simulink model "external_state_machine"  (R2021a)
settings: Solver=FixedStepDiscrete  StartTime=0.0  StopTime=2000*t_ADC  RelTol=1e-3
values from neighbouring files (symbols this model uses):
  A = 0.1    [uz_mpc_6ph_init.m]    (also in uz_mpc_6ph_state_machine_init.m)
  IB = sqrt(2)*IR    [uz_mpc_6ph_init.m]    (also in uz_mpc_6ph_state_machine_init.m)
  id_ref = 0.0    (= 0)    [uz_mpc_6ph_init.m]    (also in uz_mpc_6ph_state_machine_init.m)
  iq_ref = 15.0    (= 15)    [uz_mpc_6ph_init.m]    (also in uz_mpc_6ph_state_machine_init.m = 10)
  ix_ref = 0.0    (= 0)    [uz_mpc_6ph_init.m]    (also in uz_mpc_6ph_state_machine_init.m)
  iy_ref = 0.0    (= 0)    [uz_mpc_6ph_init.m]    (also in uz_mpc_6ph_state_machine_init.m)
  lambda_d = 1.0    (= 1)    [uz_mpc_6ph_init.m]    (also in uz_mpc_6ph_state_machine_init.m)
  lambda_q = 1.0    (= 1)    [uz_mpc_6ph_init.m]    (also in uz_mpc_6ph_state_machine_init.m)
  lambda_u = 0.0    (= 0)    [uz_mpc_6ph_init.m]    (also in uz_mpc_6ph_state_machine_init.m)
  lambda_x = 1.0    (= 1)    [uz_mpc_6ph_init.m]    (also in uz_mpc_6ph_state_machine_init.m)
  lambda_y = 1.0    (= 1)    [uz_mpc_6ph_init.m]    (also in uz_mpc_6ph_state_machine_init.m)
  Ld_over_LB = Ld/LB    [uz_mpc_6ph_init.m]    (also in uz_mpc_6ph_state_machine_init.m)
  Lq_over_LB = Lq/LB    [uz_mpc_6ph_init.m]    (also in uz_mpc_6ph_state_machine_init.m)
  n_rpm = 2200.0    (= 2200)    [uz_mpc_6ph_init.m]    (also in uz_mpc_6ph_state_machine_init.m = 100)
  omega_m = n_rpm*pi/30    (= 230.383461263)    [uz_mpc_6ph_init.m]    (also in uz_mpc_6ph_state_machine_init.m = 10.471975512)
  omegaB = nR*2*pi()/60*p    [uz_mpc_6ph_init.m]    (also in uz_mpc_6ph_state_machine_init.m)
  p = 5    [uz_mpc_6ph_init.m]    (also in uz_mpc_6ph_state_machine_init.m)
  psi_pm_over_psiB = psi_pm/psiB    [uz_mpc_6ph_init.m]    (also in uz_mpc_6ph_state_machine_init.m)
  Rs_over_ZB = Rs/ZB    [uz_mpc_6ph_init.m]    (also in uz_mpc_6ph_state_machine_init.m)
  t_ADC = 1/f_ADC    (= 1e-05)    [uz_mpc_6ph_init.m]    (also in uz_mpc_6ph_state_machine_init.m)
  t_clock = 1/f_clock    (= 1e-08)    [uz_mpc_6ph_init.m]    (also in uz_mpc_6ph_state_machine_init.m)
  Ts_times_ZB_over_Ld = Ts*ZB/Ld    [uz_mpc_6ph_init.m]    (also in uz_mpc_6ph_state_machine_init.m)
  Ts_times_ZB_over_Lq = Ts*ZB/Lq    [uz_mpc_6ph_init.m]    (also in uz_mpc_6ph_state_machine_init.m)
  Ts_times_ZB_over_Lx = Ts*ZB/Lx    [uz_mpc_6ph_init.m]    (also in uz_mpc_6ph_state_machine_init.m)
  Ts_times_ZB_over_Ly = Ts*ZB/Ly    [uz_mpc_6ph_init.m]    (also in uz_mpc_6ph_state_machine_init.m)
  v_dc = 565.0    (= 565)    [uz_mpc_6ph_init.m]    (also in uz_mpc_6ph_state_machine_init.m = 50)
  VB = sqrt(2/3)*VR    [uz_mpc_6ph_init.m]    (also in uz_mpc_6ph_state_machine_init.m)
libraries: nesl_utility x38, fl_lib x30, simulink x19, ee_lib x14, hdlsllib x4, spsAlphaBetaZerotodq0Lib x1
(part 4 of 4)

== matlab function external_state_machine/uz_vsd_6ph_30deg/VSD_6ph_30deg ==
  settings: fimath=fimath('RoundingMethod', 'Floor','OverflowAction', 'Wrap','ProductMode', 'FullPrecision', 'SumMode', 'FullPrecision')
  data: a1 input; alpha output; b1 input; c1 input; a2 input; b2 input; c2 input; beta output; x1 output; y1 output; z1 output; z2 output
function [alpha,beta,x1,y1,z1,z2] = fcn(a1,b1,c1,a2,b2,c2)


A = [fi(0,1,18,11) fi(0,1,18,11) fi(0,1,18,11) fi(0,1,18,11) fi(0,1,18,11) fi(0,1,18,11)]';

A =    2/6*[1    -0.5        -0.5        sqrt(3)/2   -sqrt(3)/2  0 ;
           0    sqrt(3)/2   -sqrt(3)/2  0.5         0.5         -1;
           1    -0.5        -0.5        -sqrt(3)/2  sqrt(3)/2   0 ;
           0    -sqrt(3)/2  sqrt(3)/2   0.5         0.5         -1;
           0.5   0.5          0.5          0           0           0 ;
           0    0           0           0.5          0.5          0.5] * [a1 b1 c1 a2 b2 c2]';

alpha = fi(A(1),1,18,11);
beta = fi(A(2),1,18,11);
x1 = fi(A(3),1,18,11);
y1 = fi(A(4),1,18,11);
z1 = fi(A(5),1,18,11);
z2 = fi(A(6),1,18,11);

== matlab function external_state_machine/cost_opt/MATLAB Function ==
  settings: fimath=fimath('RoundingMethod', 'Floor','OverflowAction', 'Wrap','ProductMode', 'FullPrecision', 'SumMode', 'FullPrecision')
  data: in input; G_next output; index input; last_optim_index input; G_prev output
function [G_next,G_prev] = get_switch_positions(in,index,last_optim_index)
%#codegen
G_next = in(index,[1 3 5 7 9 11]);
G_prev = in(last_optim_index,[1 3 5 7 9 11]);

== matlab function external_state_machine/cost_opt/iterativesearch ==
  settings: fimath=fimath('RoundingMethod', 'Floor','OverflowAction', 'Wrap','ProductMode', 'FullPrecision', 'SumMode', 'FullPrecision')
  data: index input; opt_idx output; cost input; min_costs output; opt_done output
function [opt_idx,min_costs,opt_done] = fcn(index, cost)
%#codegen

persistent cost_old
if isempty(cost_old)
    cost_old = fi(4.98,0,27,24);
end

persistent index_old
if isempty(index_old)
    index_old = uint32(1);
end

persistent opt_idx_old
if isempty(opt_idx_old)
    opt_idx_old = uint32(1);
end


if (index < 64)       
       
if (index ~= index_old)
   if (cost <= cost_old)
       opt_idx_old = index; 
       cost_old = cost;
   else
    
    
   end
   index_old = index;
end

else
       cost_old = fi(4.98,0,27,24);
end

if (index == 64)
    opt_done = true;
else
    opt_done = false;
end

min_costs = cost_old;
opt_idx = opt_idx_old;

== matlab function external_state_machine/MATLAB Function ==
  data: u input; G_opt output; opt_idx output
function [G_opt,opt_idx] = fcn(u)
%#codegen
G = [0,1,0,1,0,1,0,1,0,1,0,1;1,0,1,0,0,1,1,0,1,0,0,1;1,0,1,0,0,1,1,0,1,0,0,1;0,1,1,0,0,1,1,0,1,0,0,1;1,0,1,0,0,1,1,0,1,0,0,1;0,1,1,0,0,1,1,0,1,0,0,1;1,0,1,0,0,1,1,0,1,0,0,1;0,1,1,0,0,1,1,0,1,0,0,1;1,0,1,0,0,1,1,0,1,0,0,1;0,1,1,0,0,1,1,0,1,0,0,1;1,0,1,0,0,1,1,0,1,0,0,1;0,1,1,0,0,1,1,0,1,0,0,1;1,0,1,0,0,1,1,0,1,0,0,1;0,1,1,0,0,1,1,0,1,0,0,1;1,0,1,0,0,1,1,0,1,0,0,1;0,1,1,0,0,1,1,0,1,0,0,1;1,0,1,0,0,1,1,0,1,0,0,1;0,1,1,0,0,1,1,0,1,0,0,1;1,0,1,0,0,1,1,0,1,0,0,1;0,1,1,0,0,1,1,0,1,0,0,1;1,0,1,0,0,1,1,0,1,0,0,1;0,1,1,0,0,1,1,0,1,0,0,1;1,0,1,0,0,1,1,0,1,0,0,1;0,1,1,0,0,1,1,0,1,0,0,1;1,0,1,0,0,1,1,0,1,0,0,1;0,1,1,0,0,1,1,0,1,0,0,1;1,0,1,0,0,1,1,0,1,0,0,1;0,1,1,0,0,1,1,0,1,0,0,1;1,0,1,0,0,1,1,0,1,0,0,1;0,1,1,0,0,1,1,0,1,0,0,1;1,0,1,0,0,1,1,0,1,0,0,1;0,1,1,0,0,1,1,0,1,0,0,1;1,0,1,0,0,1,1,0,1,0,0,1;0,1,1,0,0,1,1,0,1,0,0,1;1,0,1,0,0,1,1,0,1,0,0,1;0,1,1,0,0,1,1,0,1,0,0,1;1,0,1,0,0,1,1,0,1,0,0,1;0,1,1,0,0,1,1,0,1,0,0,1;1,0,1,0,0,1,1,0,1,0,0,1;0,1,1,0,0,1,1,0,1,0,0,1;1,0,1,0,0,1,1,0,1,0,0,1;0,1,1,0,0,1,1,0,1,0,0,1;1,0,1,0,0,1,1,0,1,0,0,1;0,1,1,0,0,1,1,0,1,0,0,1;1,0,1,0,0,1,1,0,1,0,0,1;0,1,1,0,0,1,1,0,1,0,0,1;1,0,1,0,0,1,1,0,1,0,0,1;0,1,1,0,0,1,1,0,1,0,0,1;1,0,1,0,0,1,1,0,1,0,0,1;0,1,1,0,0,1,1,0,1,0,0,1;1,0,1,0,0,1,1,0,1,0,0,1;0,1,1,0,0,1,1,0,1,0,0,1;1,0,1,0,0,1,1,0,1,0,0,1;0,1,1,0,0,1,1,0,1,0,0,1;1,0,1,0,0,1,1,0,1,0,0,1;0,1,1,0,0,1,1,0,1,0,0,1;1,0,1,0,0,1,1,0,1,0,0,1;0,1,1,0,0,1,1,0,1,0,0,1;1,0,1,0,0,1,1,0,1,0,0,1;0,1,1,0,0,1,1,0,1,0,0,1;1,0,1,0,0,1,1,0,1,0,0,1;0,1,1,0,0,1,1,0,1,0,0,1;1,0,1,0,0,1,1,0,1,0,0,1;0,1,1,0,0,1,1,0,1,0,0,1;1,0,1,0,0,1,1,0,1,0,0,1;0,1,1,0,0,1,1,0,1,0,0,1;1,0,1,0,0,1,1,0,1,0,0,1;0,1,1,0,0,1,1,0,1,0,0,1;1,0,1,0,0,1,1,0,1,0,0,1;0,1,1,0,0,1,1,0,1,0,0,1;1,0,1,0,0,1,1,0,1,0,0,1;0,1,1,0,0,1,1,0,1,0,0,1;1,0,1,0,0,1,1,0,1,0,0,1;0,1,0,1,1,0,1,0,1,0,0,1;1,0,0,1,1,0,1,0,1,0,0,1;0,1,1,0,1,0,1,0,1,0,0,1;1,0,1,0,1,0,1,0,1,0,0,1;0,1,0,1,0,1,0,1,0,1,1,0;1,0,0,1,0,1,0,1,0,1,1,0;0,1,1,0,0,1,0,1,0,1,1,0;1,0,1,0,0,1,0,1,0,1,1,0;0,1,0,1,1,0,0,1,0,1,1,0;1,0,0,1,1,0,0,1,0,1,1,0;0,1,1,0,1,0,0,1,0,1,1,0;1,0,1,0,1,0,0,1,0,1,1,0;0,1,0,1,0,1,1,0,0,1,1,0;1,0,0,1,0,1,1,0,0,1,1,0;0,1,1,0,0,1,1,0,0,1,1,0;1,0,1,0,0,1,1,0,0,1,1,0;0,1,1,0,0,1,1,0,0,1,1,0;1,0,1,0,0,1,1,0,0,1,1,0;0,1,0,1,0,1,0,1,1,0,1,0;0,1,1,0,0,1,0,1,1,0,1,0;1,0,1,0,0,1,0,1,1,0,1,0;0,1,1,0,0,1,0,1,1,0,1,0;1,0,1,0,0,1,0,1,1,0,1,0;0,1,1,0,0,1,0,1,1,0,1,0;1,0,1,0,0,1,0,1,1,0,1,0;0,1,1,0,0,1,0,1,1,0,1,0;1,0,1,0,0,1,0,1,1,0,1,0;1,0,1,0,0,1,0,1,1,0,1,0];
idx = [0;28;28;27;28;27;28;27;28;27;28;27;28;27;28;27;28;27;28;27;28;27;28;27;28;27;28;27;28;27;28;27;28;27;28;27;28;27;28;27;28;27;28;27;28;27;28;27;28;27;28;27;28;27;28;27;28;27;28;27;28;27;28;27;28;27;28;27;28;27;28;27;28;29;30;31;32;33;34;35;36;37;38;39;40;41;42;43;44;43;44;49;51;52;51;52;51;52;51;52;52];


G_opt = G(u,:);
opt_idx = idx(u);

== matlab function external_state_machine/6ph_PMSM_30deg_VSD1 ==
  data: u1 input; y1 output; u2 input; u3 input; u4 input; u5 input; u6 input; y2 output; y3 output; y4 output; y5 output; y6 output; k6 input; c6 input
function [y1,y2,y3,y4,y5,y6] = VSD_asymm_30(u1,u2,u3,u4,u5,u6,k6,c6)

A = [0 0 0 0 0 0]';

A =    k6*[1    -0.5        -0.5        sqrt(3)/2   -sqrt(3)/2  0 ;
           0    sqrt(3)/2   -sqrt(3)/2  0.5         0.5         -1;
           1    -0.5        -0.5        -sqrt(3)/2  sqrt(3)/2   0 ;
           0    -sqrt(3)/2  sqrt(3)/2   0.5         0.5         -1;
           c6   c6          c6          0           0           0 ;
           0    0           0           c6          c6          c6] * [u1 u2 u3 u4 u5 u6]';

y1 = A(1);
y2 = A(2);
y3 = A(3);
y4 = A(4);
y5 = A(5);
y6 = A(6);

== matlab function external_state_machine/cost_opt/FiniteControlSetSwitchingTable ==
  settings: fimath=fimath('RoundingMethod', 'Floor','OverflowAction', 'Wrap','ProductMode', 'FullPrecision', 'SumMode', 'FullPrecision')
  data: G output
function G  = switchingTable

% -------------------------------------------------------------------
%  Generated by MATLAB on 14-Oct-2020 14:52:37
%  MATLAB version: 9.4.0.813654 (R2018a)
% -------------------------------------------------------------------
                                         

s1_v = boolean([0; 1; 0; 1; 0; 1; 0; 1; 0; 1; 0; 1; 0; 1; 0; 1; 0; 1; 0; 1; 0; ...
        1; 0; 1; 0; 1; 0; 1; 0; 1; 0; 1; 0; 1; 0; 1; 0; 1; 0; 1; 0; 1; ...
        0; 1; 0; 1; 0; 1; 0; 1; 0; 1; 0; 1; 0; 1; 0; 1; 0; 1; 0; 1; 0; ...
        1]);


s2_v = boolean([1; 0; 1; 0; 1; 0; 1; 0; 1; 0; 1; 0; 1; 0; 1; 0; 1; 0; 1; 0; 1; ...
        0; 1; 0; 1; 0; 1; 0; 1; 0; 1; 0; 1; 0; 1; 0; 1; 0; 1; 0; 1; 0; ...
        1; 0; 1; 0; 1; 0; 1; 0; 1; 0; 1; 0; 1; 0; 1; 0; 1; 0; 1; 0; 1; ...
        0]);


s3_v = boolean([0; 0; 1; 1; 0; 0; 1; 1; 0; 0; 1; 1; 0; 0; 1; 1; 0; 0; 1; 1; 0; ...
        0; 1; 1; 0; 0; 1; 1; 0; 0; 1; 1; 0; 0; 1; 1; 0; 0; 1; 1; 0; 0; ...
        1; 1; 0; 0; 1; 1; 0; 0; 1; 1; 0; 0; 1; 1; 0; 0; 1; 1; 0; 0; 1; ...
        1]);


s4_v = boolean([1; 1; 0; 0; 1; 1; 0; 0; 1; 1; 0; 0; 1; 1; 0; 0; 1; 1; 0; 0; 1; ...
        1; 0; 0; 1; 1; 0; 0; 1; 1; 0; 0; 1; 1; 0; 0; 1; 1; 0; 0; 1; 1; ...
        0; 0; 1; 1; 0; 0; 1; 1; 0; 0; 1; 1; 0; 0; 1; 1; 0; 0; 1; 1; 0; ...
        0]);


s5_v = boolean([0; 0; 0; 0; 1; 1; 1; 1; 0; 0; 0; 0; 1; 1; 1; 1; 0; 0; 0; 0; 1; ...
        1; 1; 1; 0; 0; 0; 0; 1; 1; 1; 1; 0; 0; 0; 0; 1; 1; 1; 1; 0; 0; ...
        0; 0; 1; 1; 1; 1; 0; 0; 0; 0; 1; 1; 1; 1; 0; 0; 0; 0; 1; 1; 1; ...
        1]);


s6_v = boolean([1; 1; 1; 1; 0; 0; 0; 0; 1; 1; 1; 1; 0; 0; 0; 0; 1; 1; 1; 1; 0; ...
        0; 0; 0; 1; 1; 1; 1; 0; 0; 0; 0; 1; 1; 1; 1; 0; 0; 0; 0; 1; 1; ...
        1; 1; 0; 0; 0; 0; 1; 1; 1; 1; 0; 0; 0; 0; 1; 1; 1; 1; 0; 0; 0; ...
        0]);


s7_v = boolean([0; 0; 0; 0; 0; 0; 0; 0; 1; 1; 1; 1; 1; 1; 1; 1; 0; 0; 0; 0; 0; ...
        0; 0; 0; 1; 1; 1; 1; 1; 1; 1; 1; 0; 0; 0; 0; 0; 0; 0; 0; 1; 1; ...
        1; 1; 1; 1; 1; 1; 0; 0; 0; 0; 0; 0; 0; 0; 1; 1; 1; 1; 1; 1; 1; ...
        1]);


s8_v = boolean([1; 1; 1; 1; 1; 1; 1; 1; 0; 0; 0; 0; 0; 0; 0; 0; 1; 1; 1; 1; 1; ...
        1; 1; 1; 0; 0; 0; 0; 0; 0; 0; 0; 1; 1; 1; 1; 1; 1; 1; 1; 0; 0; ...
        0; 0; 0; 0; 0; 0; 1; 1; 1; 1; 1; 1; 1; 1; 0; 0; 0; 0; 0; 0; 0; ...
        0]);


s9_v = boolean([0; 0; 0; 0; 0; 0; 0; 0; 0; 0; 0; 0; 0; 0; 0; 0; 1; 1; 1; 1; 1; ...
        1; 1; 1; 1; 1; 1; 1; 1; 1; 1; 1; 0; 0; 0; 0; 0; 0; 0; 0; 0; 0; ...
        0; 0; 0; 0; 0; 0; 1; 1; 1; 1; 1; 1; 1; 1; 1; 1; 1; 1; 1; 1; 1; ...
        1]);


s10_v = boolean([1; 1; 1; 1; 1; 1; 1; 1; 1; 1; 1; 1; 1; 1; 1; 1; 0; 0; 0; 0; 0; ...
         0; 0; 0; 0; 0; 0; 0; 0; 0; 0; 0; 1; 1; 1; 1; 1; 1; 1; 1; 1; 1; ...
         1; 1; 1; 1; 1; 1; 0; 0; 0; 0; 0; 0; 0; 0; 0; 0; 0; 0; 0; 0; 0; ...
         0]);


s11_v = boolean([0; 0; 0; 0; 0; 0; 0; 0; 0; 0; 0; 0; 0; 0; 0; 0; 0; 0; 0; 0; 0; ...
         0; 0; 0; 0; 0; 0; 0; 0; 0; 0; 0; 1; 1; 1; 1; 1; 1; 1; 1; 1; 1; ...
         1; 1; 1; 1; 1; 1; 1; 1; 1; 1; 1; 1; 1; 1; 1; 1; 1; 1; 1; 1; 1; ...
         1]);


s12_v = boolean([1; 1; 1; 1; 1; 1; 1; 1; 1; 1; 1; 1; 1; 1; 1; 1; 1; 1; 1; 1; 1; ...
         1; 1; 1; 1; 1; 1; 1; 1; 1; 1; 1; 0; 0; 0; 0; 0; 0; 0; 0; 0; 0; ...
         0; 0; 0; 0; 0; 0; 0; 0; 0; 0; 0; 0; 0; 0; 0; 0; 0; 0; 0; 0; 0; ...
         0]);
     
G = [s1_v, s2_v, s3_v, s4_v, s5_v, s6_v, s7_v, s8_v, s9_v, s10_v, s11_v, s12_v];

== matlab function external_state_machine/Subsystem2/Count_f_sw ==
  data: switchNumb input fixdt(0,25,0); ss_v_old input; ss_v input; switchNumbOut output fixdt(0,25,0); bReset input
 function switchNumbOut   = Count_f_sw(switchNumb,ss_v_old,ss_v, bReset)
   %
    %% toDO
        %s
 
    %% Initialization
    Fq25    = fimath('RoundingMethod', 'Floor', 'OverflowAction', 'Wrap','ProductMode', 'FullPrecision', 'ProductWordLength', 25,'ProductFractionLength',0,'SumMode','SpecifyPrecision','SumWordLength',25,'SumFractionLength',0);

    % I need this initialization, in order that the HDL Coder and Simulink knows the size of the vectors! Without these, i will get an error!
   % idx_globalOld     = fi(1, 0, 8, 0); % Chosen position overall in the error vector
    %switchNumb = fi(0, 0, 25, 0);
    
    %% Reset the counters (similar to the THD, i will try to average the switching frequency over 20 fundamental periods. After this time, a Reset-Flag from the ARM processor will reset the counter) 
    if (bReset == true) 
        switchNumb = fi(0, 0, 25, 0);
    end
    %% Check if switching occurs. If yes count up.
    % However, dependent of the ss_v before, switching can but do not have to occure, if the previously applied ss_v keeps.

    %Use a for-loop since in VHDL i have time and can do a resource streaming
    %Even if i need 6 cycles @100MHz, since it is not able to have have
    %switching (on/off inside of 60ns), this is ok (because T_cf = 10us and
    %and switching for such a short time is not allwoed nayway, since it is
    %not worth it (too much losses).)
    for countSS=fi(1, 0, 8, 0):fi(12, 0, 8, 0) %1:12
        if (ss_v(countSS) ~= ss_v_old(countSS)) %Check if switch has changed
            switchNumb = fi(add(Fq25,switchNumb,fi(1, 0, 25, 0)),0,25,0); % +1 Increment the switch counter +1
        end
    end

    switchNumbOut = switchNumb;

 end
